simulink model "part2controller"  (R2021b)
settings: Solver=VariableStepAuto  StartTime=0.0  StopTime=10.0  RelTol=1e-3
model workspace (MAT data in the model file):
  Kp = 0.15
settings Model: Creator=parth  LastModifiedBy=parth

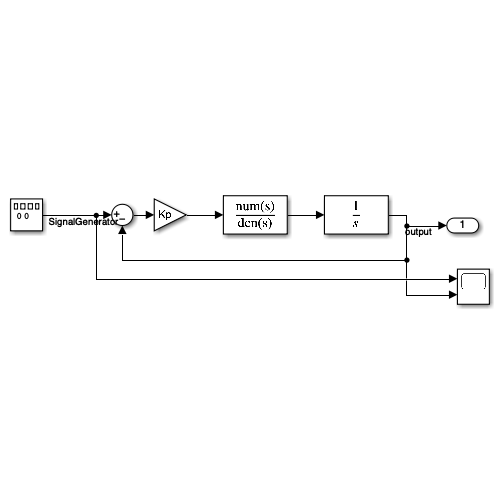
[thumbnail: Simulink's stored preview of the top-level diagram]
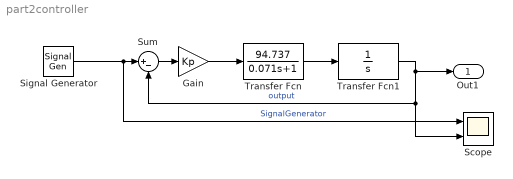
== system part2controller ==
  Gain : Gain  Gain=Kp
  Scope : Scope  NumInputPorts=2
  Signal Generator : SignalGenerator  WaveForm=square  Amplitude=5  Frequency=0.5
  Sum : Sum  Inputs=|+-
  Transfer Fcn : TransferFcn  Numerator=[94.737]  Denominator=[0.071 1]
  Transfer Fcn1 : TransferFcn  Denominator=[1 0]
  Out1 : Outport
  wires:
  Gain/1 -> Transfer Fcn/1
  Transfer Fcn/1 -> Transfer Fcn1/1
  Transfer Fcn1/1 -> Out1/1, Sum/2, Scope/2  "output"
  Signal Generator/1 -> Scope/1, Sum/1  "SignalGenerator"
  Sum/1 -> Gain/1
